simulink model "servoIdent"  (R2015b)
settings: Solver=ode3  SolverMode=SingleTasking  StartTime=0.0  StopTime=inf  RelTol=1e-3
undefined symbols (not defined in the file or in its folder): DiscIntNeverNeededParam
libraries: arduino_io_lib x5, simulink x1, dspfdesign x1, slident x1
settings Model: ExtModeTrigDuration=2  Creator=gcampa  LastModifiedBy=Jack
settings DataIOCC: SaveFormat=Array
settings OptimizationCC: OptimizeModelRefInitCode=on  LifeSpan=1  MaxStackSize=64
settings DebuggingCC: UnderspecifiedInitializationDetection=Classic  MergeDetectMultiDrivingBlocksExec=none
settings HardwareCC: ProdBitPerInt=16  ProdBitPerPointer=16  ProdLargestAtomicFloat=None  ProdWordSize=8  ProdHWDeviceType=Atmel->AVR
settings RTWCC: SystemTargetFile=ert.tlc  TemplateMakefile=ert_default_tmf  Description=Embedded Coder  RTWVerbose=off  Toolchain=Arduino AVR v1.6.1  BuildConfiguration=Faster Runs
settings CodeAppCC: IgnoreCustomStorageClasses=off
settings ERTTargetCC: SupportContinuousTime=on  SupportVariableSizeSignals=on
settings ConfigComp: CovModelRefEnable=Off

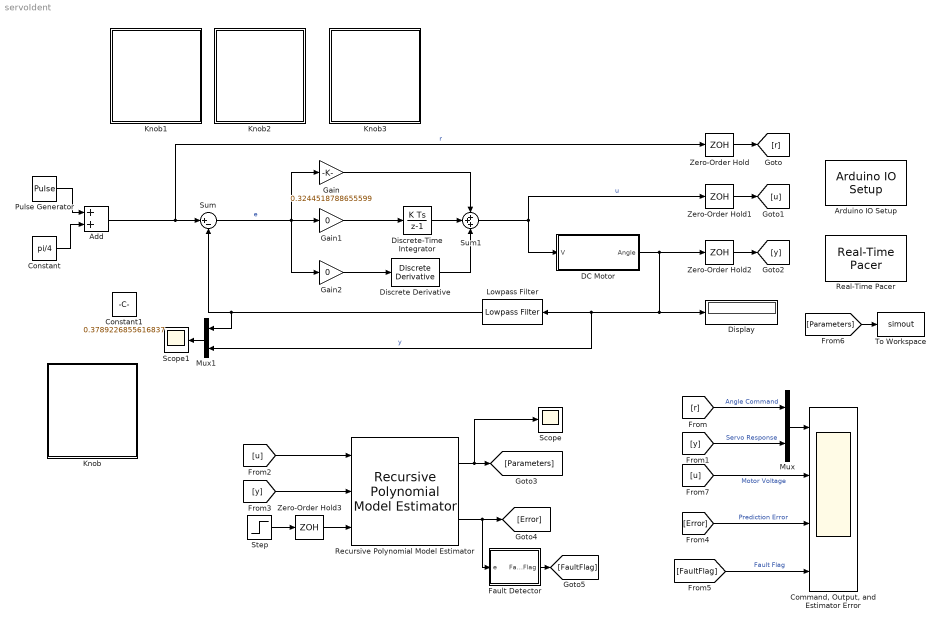
== system servoIdent ==
  Add : Sum
  Arduino IO Setup : arduino_io_lib/Arduino IO Setup  Priority=3  arduinoVar=Temporary arduino variable: Arduino1  workspaceVarName=b  comPort=/dev/tty.usbmodemFA131
  "Command, Output, and Estimator Error" : Scope  NumInputPorts=4
  Constant : Constant  Value=pi/4
  Constant1 : Constant  Value=0.3789226855616837
  DC Motor : Subsystem
  Discrete Derivative : simulink/Discrete/Discrete Derivative  gainval=1.0  ICPrevScaledInput=0.0  InputProcessing=Inherited  OutMin=[]  OutMax=[]  OutDataType=fixdt(1, 16)  OutScaling=2^-10  DoSatur=off
  Discrete-Time Integrator : DiscreteIntegrator  InitialConditionSetting=State (most efficient)  ICPrevOutput=DiscIntNeverNeededParam  ICPrevScaledInput=DiscIntNeverNeededParam
  Display : Display
  Fault Detector : Subsystem
  Gain : Gain  Gain=0.3244518788655599
  Gain1 : Gain  Gain=0
  Gain2 : Gain  Gain=0
  Knob : Subsystem  DialogController=hmiCreateDDGDialog  IsWebBlock=on  mask(MWDashboardBlock){webBlockId=445a0260-38bd-4b17-b971-db3368aaab99, webBlockType=continuousknob, ShowInLibBrowser=on, ShowInitialText=on, HMISrcModelName=servoIdent}
      mask prompts: webBlockId "WebBlock Id"; webBlockType "WebBlock Type"; HMISrcModelName "Source Model"
      mask Help: helpview([docroot '/mapfiles/simulink.map'], 'hmi_knob')
      mask Display:
      | if strcmp(get_param(bdroot(gcb),'BlockDiagramType'), 'library')
      |     image([(matlabroot) '/toolbox/simulink/hmi/icons/ContinuousKnob.png']);
      | end
  Knob1 : Subsystem  DialogController=hmiCreateDDGDialog  IsWebBlock=on  mask(MWDashboardBlock){webBlockId=12bbddad-4295-43db-befe-2cc76af55062, webBlockType=continuousknob, ShowInLibBrowser=on, ShowInitialText=on, HMISrcModelName=servoIdent}
      mask prompts: webBlockId "WebBlock Id"; webBlockType "WebBlock Type"; HMISrcModelName "Source Model"
      mask Help: helpview([docroot '/mapfiles/simulink.map'], 'hmi_knob')
      mask Display:
      | if strcmp(get_param(bdroot(gcb),'BlockDiagramType'), 'library')
      |     image([(matlabroot) '/toolbox/simulink/hmi/icons/ContinuousKnob.png']);
      | end
  Knob2 : Subsystem  DialogController=hmiCreateDDGDialog  IsWebBlock=on  mask(MWDashboardBlock){webBlockId=60666d6e-d21d-4047-8675-97cd4ac2fe9f, webBlockType=continuousknob, ShowInLibBrowser=on, ShowInitialText=on, HMISrcModelName=servoIdent}
      mask prompts: webBlockId "WebBlock Id"; webBlockType "WebBlock Type"; HMISrcModelName "Source Model"
      mask Help: helpview([docroot '/mapfiles/simulink.map'], 'hmi_knob')
      mask Display:
      | if strcmp(get_param(bdroot(gcb),'BlockDiagramType'), 'library')
      |     image([(matlabroot) '/toolbox/simulink/hmi/icons/ContinuousKnob.png']);
      | end
  Knob3 : Subsystem  DialogController=hmiCreateDDGDialog  IsWebBlock=on  mask(MWDashboardBlock){webBlockId=b5b8342f-5a5b-4bd1-b163-81508368278c, webBlockType=continuousknob, ShowInLibBrowser=on, ShowInitialText=on, HMISrcModelName=servoIdent}
      mask prompts: webBlockId "WebBlock Id"; webBlockType "WebBlock Type"; HMISrcModelName "Source Model"
      mask Help: helpview([docroot '/mapfiles/simulink.map'], 'hmi_knob')
      mask Display:
      | if strcmp(get_param(bdroot(gcb),'BlockDiagramType'), 'library')
      |     image([(matlabroot) '/toolbox/simulink/hmi/icons/ContinuousKnob.png']);
      | end
  Lowpass Filter : dspfdesign/Lowpass Filter  FilterType=FIR  DesignForMinimumOrder=on  FilterOrder=50  PassbandFrequency=8e3  StopbandFrequency=12e3  PassbandRipple=0.1  StopbandAttenuation=80  InheritSampleRate=off  SampleRate=44100  roundingMode=Floor  coeffsDataTypeStr=fixdt(1,16)  SimulateUsing=Interpreted execution
  Mux : Mux  Inputs=2
  Mux1 : Mux  Inputs=2
  Pulse Generator : DiscretePulseGenerator  PulseType=Time based  Amplitude=pi/2  Period=8  PulseWidth=50
  Real-Time Pacer : arduino_io_lib/Real-Time Pacer  simTimePerRealTime=1
  Recursive Polynomial Model Estimator : slident/Estimators/Recursive Polynomial Model Estimator  ModelStructure=ARMAX  InitialEstimateSource=None  A0=2  B0=2  C0=1  D0=1  F0=1  nk=2  P0=1e4  EstimationMethod=Forgetting Factor  AdaptationParameter=1  NormalizationBias=eps  OutputError=on  OutputP=off  AddEnablePort=on  Ts=-1
  Scope : Scope
  Scope1 : Scope
  Step : Step  Time=15  Before=1  After=0  SampleTime=0
  Sum : Sum  Inputs=|+-
  Sum1 : Sum  Inputs=+++
  To Workspace : ToWorkspace  VariableName=simout  SaveFormat=Timeseries  SampleTime=-1
  Zero-Order Hold{,1..3} (4 alike) : ZeroOrderHold  SampleTime=1/200
  wires:
  Add/1 -> Zero-Order Hold/1, Sum/1  "r"
  Constant/1 -> Add/2
  Pulse Generator/1 -> Add/1
  DC Motor/1(Angle) -> Zero-Order Hold2/1, Mux1/2, Lowpass Filter/1, Display/1  "y"
  Sum1/1 -> DC Motor/1(V), Zero-Order Hold1/1  "u"
  [y] -> Mux/2  "Servo Response"
  [r] -> Mux/1  "Angle Command"
  [u] -> Recursive Polynomial Model Estimator/1
  [y] -> Recursive Polynomial Model Estimator/2
  Recursive Polynomial Model Estimator/1 -> Scope/1, [Parameters]
  Recursive Polynomial Model Estimator/2 -> Fault Detector/1(e), [Error]
  [Error] -> "Command, Output, and Estimator Error"/3  "Prediction Error"
  Zero-Order Hold/1 -> [r]
  Zero-Order Hold1/1 -> [u]
  Zero-Order Hold2/1 -> [y]
  Fault Detector/1(FaultFlag) -> [FaultFlag]
  [FaultFlag] -> "Command, Output, and Estimator Error"/4  "Fault Flag"
  Step/1 -> Zero-Order Hold3/1
  Zero-Order Hold3/1 -> Recursive Polynomial Model Estimator/3
  Sum/1 -> Gain2/1, Gain1/1, Gain/1  "e"
  [Parameters] -> To Workspace/1
  [u] -> "Command, Output, and Estimator Error"/2  "Motor Voltage"
  Mux/1 -> "Command, Output, and Estimator Error"/1
  Mux1/1 -> Scope1/1
  Lowpass Filter/1 -> Mux1/1, Sum/2
  Gain1/1 -> Discrete-Time Integrator/1
  Discrete-Time Integrator/1 -> Sum1/2
  Discrete Derivative/1 -> Sum1/3
  Gain/1 -> Sum1/1
  Gain2/1 -> Discrete Derivative/1

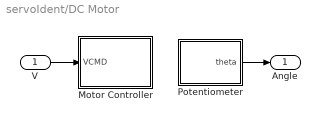
== system servoIdent/DC Motor ==
  V : Inport
  Motor Controller : Subsystem
  Potentiometer : Subsystem
  Angle : Outport
  wires:
  V/1 -> Motor Controller/1(VCMD)
  Potentiometer/1(theta) -> Angle/1

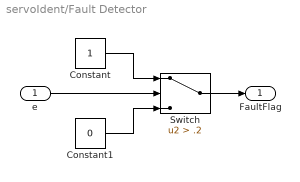
== system servoIdent/Fault Detector ==
  e : Inport
  Constant : Constant
  Constant1 : Constant  Value=0
  Switch : Switch  Criteria=u2 > Threshold  Threshold=.2
  FaultFlag : Outport
  wires:
  Switch/1 -> FaultFlag/1
  e/1 -> Switch/2
  Constant/1 -> Switch/1
  Constant1/1 -> Switch/3

== system servoIdent/Knob ==

== system servoIdent/Knob1 ==

== system servoIdent/Knob2 ==

== system servoIdent/Knob3 ==

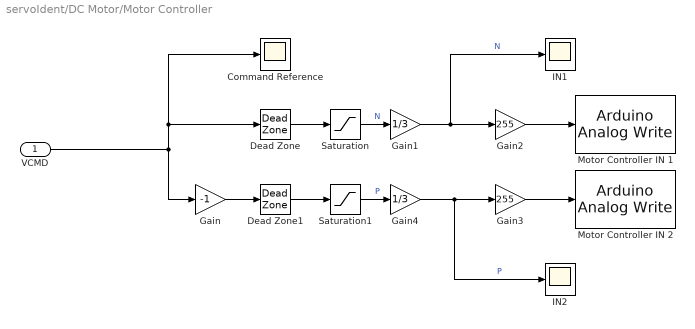
== system servoIdent/DC Motor/Motor Controller ==
  VCMD : Inport
  Command Reference : Scope
  Dead Zone : DeadZone  LowerValue=-inf  UpperValue=0  SaturateOnIntegerOverflow=on
  Dead Zone1 : DeadZone  LowerValue=-inf  UpperValue=0  SaturateOnIntegerOverflow=on
  Gain : Gain  Gain=-1
  Gain1 : Gain  Gain=1/3
  Gain2 : Gain  Gain=255
  Gain3 : Gain  Gain=255
  Gain4 : Gain  Gain=1/3
  IN1 : Scope
  IN2 : Scope
  Motor Controller IN 1 : arduino_io_lib/Arduino Analog Write  arduinoVar=Temporary arduino variable: Arduino1  arduinoPin=3  T=0.2
  "Motor Controller IN 2 " : arduino_io_lib/Arduino Analog Write  arduinoVar=Temporary arduino variable: Arduino1  arduinoPin=2  T=0.2
  Saturation : Saturate  UpperLimit=3  LowerLimit=0
  Saturation1 : Saturate  UpperLimit=3  LowerLimit=0
  wires:
  Dead Zone/1 -> Saturation/1
  VCMD/1 -> Command Reference/1, Dead Zone/1, Gain/1
  Gain1/1 -> Gain2/1, IN1/1  "N"
  Gain/1 -> Dead Zone1/1
  Dead Zone1/1 -> Saturation1/1
  Gain4/1 -> Gain3/1, IN2/1  "P"
  Gain2/1 -> Motor Controller IN 1/1
  Gain3/1 -> "Motor Controller IN 2 "/1
  Saturation/1 -> Gain1/1  "N"
  Saturation1/1 -> Gain4/1  "P"

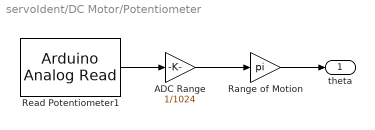
== system servoIdent/DC Motor/Potentiometer ==
  ADC Range : Gain  Gain=1/1024
  Range of Motion : Gain  Gain=pi
  Read Potentiometer1 : arduino_io_lib/Arduino Analog Read  arduinoVar=Temporary arduino variable: Arduino1  arduinoPin=0  T=0.01
  theta : Outport
  wires:
  Range of Motion/1 -> theta/1
  Read Potentiometer1/1 -> ADC Range/1
  ADC Range/1 -> Range of Motion/1
